simulink model "OpencircuitSaturation"  (Simulink 7.6)
settings: Solver=ode45  StartTime=0.0  StopTime=0.2  RelTol=1e-3
libraries: powerlib x10
settings Model: Creator=Martine  LastModifiedBy=ROOTS

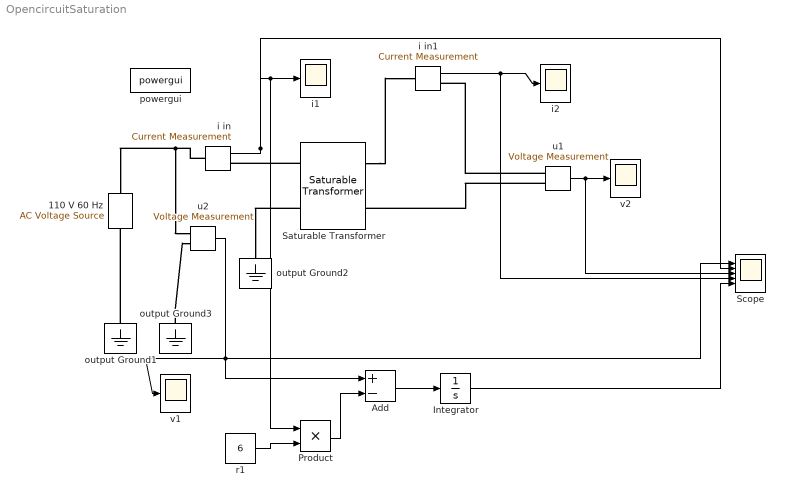
== system OpencircuitSaturation ==
  110 V 60 Hz : powerlib/Electrical Sources/AC Voltage Source  Description=source block  DialogController=POWERSYS.PowerSysDialog  SystemSampleTime=-1  Amplitude=155.563  Phase=0  Frequency=60  SampleTime=0  Measurements=None
      settings: AttributesFormatString=\n
  Add : Sum  Inputs=+-
  Integrator : Integrator
  Product : Product  RndMeth=Zero
  Saturable Transformer : powerlib/Elements/Saturable Transformer  DialogController=POWERSYS.PowerSysDialog  SystemSampleTime=-1  ThreeWindings=off  UNITS=SI  NominalPower=[75e3,60]  Winding1=[110 6 0.0135]  Winding2=[110 5 0.0135]  Winding3=[3.15e+005 2646 280.75]  Saturation=|  CoreLoss=[99.5 0.2639]  Hysteresis=off  DataFile='hysteresis.mat'  Measurements=All measurements (V I Flux)  MoreParameters=off  BreakLoop=off  DataType=on  InitialFlux=-0.38827221820321  TransfoNumber=1
      | [0,0;0.3788,0.1;0.5144,0.1374;0.7165,0.194;0.8267,0.216;1.0769,0.2457;1.3778,0.2805
      | ;1.6648,0.30624;2.1057,0.33624;2.774,0.3374;3.4905,0.3778;4.3649,0.4089;5.273,0.469
      | ;6.11,0.474;7.04,0.476;7.95,0.476;8.427,0.476;9.48,0.476]
  Scope : Scope  NumInputPorts=5
      settings: DeleteFcn=simscope BlockIsBeingDestroyed  PostSaveFcn=simscope Save  TickLabels=on  TimeRange=0.2  YMin=-200~-5~-5~-5~-5  YMax=200~5~5~5~5  SaveName=ScopeData4  DataFormat=Array
  i in : powerlib/Measurements/Current Measurement  Tag=PoWeRsYsTeMmEaSuReMeNt  DialogController=POWERSYS.PowerSysDialog  SystemSampleTime=-1  PhasorSimulation=off  OutputType=Magnitude  PSBequivalent=0
  i in1 : powerlib/Measurements/Current Measurement  Tag=PoWeRsYsTeMmEaSuReMeNt  DialogController=POWERSYS.PowerSysDialog  SystemSampleTime=-1  PhasorSimulation=off  OutputType=Magnitude  PSBequivalent=0
  i1 : Scope
      settings: DeleteFcn=simscope BlockIsBeingDestroyed  PostSaveFcn=simscope Save  TickLabels=on  TimeRange=0.1  YMin=-12.5  YMax=12.5  SaveName=ScopeData3  DataFormat=Array
  i2 : Scope
      settings: DeleteFcn=simscope BlockIsBeingDestroyed  PostSaveFcn=simscope Save  TickLabels=on  TimeRange=0.1  YMin=-12.5  YMax=12.5  SaveName=ScopeData2  DataFormat=Array
  output Ground1 : powerlib/Elements/Ground  DialogController=POWERSYS.PowerSysDialog  PhysicalDomain=powersysdomain  SubClassName=unknown  LeftPortType=p1  RightPortType=p1  LConnTagsString=a
  output Ground2 : powerlib/Elements/Ground  DialogController=POWERSYS.PowerSysDialog  PhysicalDomain=powersysdomain  SubClassName=unknown  LeftPortType=p1  RightPortType=p1  LConnTagsString=a
  output Ground3 : powerlib/Elements/Ground  DialogController=POWERSYS.PowerSysDialog  PhysicalDomain=powersysdomain  SubClassName=unknown  LeftPortType=p1  RightPortType=p1  LConnTagsString=a
  powergui : powerlib/powergui  SystemSampleTime=-1  SimulationMode=Continuous  SampleTime=0  frequency=60  SPID=off  DisableSnubberDevices=off  DisableRonSwitches=off  DisableVfSwitches=off  SwTol=0  Interpol=off  frequencyindice=60  echomessages=off  HookPort=off  DisplayEquations=off  FunctionMessages=off  EnableUseOfTLC=off  x0status=blocks  RestoreLinks=warning  ResistiveCurrentMeasurement=off  Frange=[0:2:500]  Ylog=off  Xlog=on  ShowGrid=off  save=off  variable=ZData  ZoomFFT=on  StartTime=0.0  cycles=1  DisplayStyle=1  fundamental=60  FreqAxis=off  MaxFrequency=1000  frequencyindicesteady=1  RmsSteady=1  display=off  Ts=0  methode=off
  r1 : Constant  Value=6
  u1 : powerlib/Measurements/Voltage Measurement  Tag=PoWeRsYsTeMmEaSuReMeNt  DialogController=POWERSYS.PowerSysDialog  SystemSampleTime=-1  PhasorSimulation=off  OutputType=Magnitude  PSBequivalent=0
  u2 : powerlib/Measurements/Voltage Measurement  Tag=PoWeRsYsTeMmEaSuReMeNt  DialogController=POWERSYS.PowerSysDialog  SystemSampleTime=-1  PhasorSimulation=off  OutputType=Magnitude  PSBequivalent=0
  v1 : Scope
      settings: DeleteFcn=simscope BlockIsBeingDestroyed  PostSaveFcn=simscope Save  TickLabels=on  TimeRange=0.1  YMin=-200  YMax=200  DataFormat=Array
  v2 : Scope
      settings: DeleteFcn=simscope BlockIsBeingDestroyed  PostSaveFcn=simscope Save  TickLabels=on  TimeRange=0.1  YMin=-200  YMax=200  DataFormat=Array
  wires:
  u1/1 -> v2/1, Scope/3
  u2/1 -> Scope/1, Add/1, v1/1
  i in1/1 -> i2/1, Scope/4
  i in/1 -> i1/1, Product/1, Scope/2
  r1/1 -> Product/2
  Product/1 -> Add/2
  Integrator/1 -> Scope/5
  Add/1 -> Integrator/1
  connections:
  i in/LConn1 -- 110 V 60 Hz/RConn1 -- u2/LConn1
  output Ground1/LConn1 -- 110 V 60 Hz/LConn1
  output Ground3/LConn1 -- u2/LConn2
  Saturable Transformer/RConn1 -- i in1/LConn1
  u1/LConn1 -- i in1/RConn1
  Saturable Transformer/LConn1 -- i in/RConn1
  Saturable Transformer/LConn2 -- output Ground2/LConn1
  u1/LConn2 -- Saturable Transformer/RConn2
